simulink model "Duke_Simulink_13a"  (R2013a)
settings: Solver=FixedStepDiscrete  StartTime=0  StopTime=tempoSimulacao  FixedStep=1  RelTol=1e-3
values from neighbouring files (symbols this model uses):
  Ajustes_Inicial = dadosNumeroConstantes(linha)    [read_parametros_v2.m]
  aliquotaIR = dadosNumeroConstantes(linha)    [read_parametros_v2.m]
  CaixaInicial = dadosNumeroConstantes(linha)    [read_parametros_v2.m]
  Capital_Social_Inicial = CapitalSocial(1,2:end)    [Duke_main_v2.m]
  CFURH = dadosNumeroConstantes(linha)*TAR    [read_parametros_v2.m]
  contribuicaoCCEE = dadosNumeroConstantes(linha)    [read_parametros_v2.m]
  deducaoP_D = dadosNumeroConstantes(linha)    [read_parametros_v2.m]
  den_Ajustes = [1 zeros(1,PeriodoDepreciacao_Ajustes)]    [gera_Input_modelo.m]
  den_CustoAnual = [1 zeros(1,PeriodoCustoAnual-1)]    [gera_Input_modelo.m]
  den_CustoSemestral = [1 zeros(1,PeriodoCustoSemestral-1)]    [gera_Input_modelo.m]
  den_PPE_Edificacoes = [1 zeros(1,PPE_Periodo_Edificacoes)]    [gera_Input_modelo.m]
  den_PPE_Maquinas = [1 zeros(1,PPE_Periodo_Maquinas)]    [gera_Input_modelo.m]
  den_PPE_Moveis = [1 zeros(1,PPE_Periodo_Moveis)]    [gera_Input_modelo.m]
  den_PPE_Reservatorio = [1 zeros(1,PPE_Periodo_Reservatorio)]    [gera_Input_modelo.m]
  den_PPE_Veiculos = [1 zeros(1,PPE_Periodo_Veiculos)]    [gera_Input_modelo.m]
  DividaInicial = MtM_Total_Dividas(1,2:end)    [Duke_main_v2.m]
  Dividendos_A_Pagar_Inicial = dadosNumeroConstantes(linha)    [read_parametros_v2.m]
  garantiaFisica = dadosNumeroConstantes(linha)    [read_parametros_v2.m]
  IC_DividendosAPagarInicial = [repmat(vetor_DividendosAPagarInicial(1),numRealidades,1); zeros(realidadesPorSimulacao-numRealidades,1)]    [gera_Input_modelo.m]
  inicializa_JSCP = zeros(realidadesPorSimulacao,mes_JSCP)    [Duke_main_v2.m]
  IR_diferido_acumulado_inicial = dadosNumeroConstantes(linha)    [read_parametros_v2.m]
  JSCP_A_Pagar_Inicial = dadosNumeroConstantes(linha)    [read_parametros_v2.m]
  JSCP_ParcialPeriodo = dadosNumeroConstantes(linha)    [read_parametros_v2.m]
  JSCP_RetidoInicial = 0    [Duke_main_v2.m]
  Limite_Reserva_Lucros = dadosNumeroConstantes(linha)    [read_parametros_v2.m]
  Limite_Reserva_Lucros_Capital = dadosNumeroConstantes(linha)    [read_parametros_v2.m]
  LucroParcialPeriodo = dadosNumeroConstantes(linha)    [read_parametros_v2.m]
  LucroRetidoInicial = dadosNumeroConstantes(linha)    [read_parametros_v2.m]
  mes_DataInicial = month(DataInicial)    [Duke_main_v2.m]
  mes_JSCP = dadosNumeroConstantes(linha)    [read_parametros_v2.m]
  num_Ajustes = [0 ones(1,PeriodoDepreciacao_Ajustes)]*(1/PeriodoDepreciacao_Ajustes)    [gera_Input_modelo.m]
  num_CustoAnual = ones(1,PeriodoCustoAnual)*(1/PeriodoCustoAnual)    [gera_Input_modelo.m]
  num_CustoSemestral = ones(1,PeriodoCustoSemestral)*(1/PeriodoCustoSemestral)    [gera_Input_modelo.m]
  num_PPE_Edificacoes = [0 ones(1,PPE_Periodo_Edificacoes)]*(1/PPE_Periodo_Edificacoes)    [gera_Input_modelo.m]
  num_PPE_Maquinas = [0 ones(1,PPE_Periodo_Maquinas)]*(1/PPE_Periodo_Maquinas)    [gera_Input_modelo.m]
  num_PPE_Moveis = [0 ones(1,PPE_Periodo_Moveis)]*(1/PPE_Periodo_Moveis)    [gera_Input_modelo.m]
  num_PPE_Reservatorio = [0 ones(1,PPE_Periodo_Reservatorio)]*(1/PPE_Periodo_Reservatorio)    [gera_Input_modelo.m]
  num_PPE_Veiculos = [0 ones(1,PPE_Periodo_Veiculos)]*(1/PPE_Periodo_Veiculos)    [gera_Input_modelo.m]
  Outros_Passivos = dadosNumeroConstantes(linha)    [read_parametros_v2.m]
  periodoDividendos = dadosNumeroConstantes(linha)    [read_parametros_v2.m]
  periodoDividendos_delay = periodoDividendos    [Duke_main_v2.m]
  PeriodoIR_diferido = 12    [Duke_main_v2.m]
  PeriodoJSCP = 12    [Duke_main_v2.m]
  PIS_COFINS_Cumulativo = PIS + COFINS    [read_parametros_v2.m]
  PPE_Inicial_Edificacoes = dadosNumeroConstantes(linha)    [read_parametros_v2.m]
  PPE_Inicial_Maquinas = dadosNumeroConstantes(linha)    [read_parametros_v2.m]
  PPE_Inicial_Moveis = dadosNumeroConstantes(linha)    [read_parametros_v2.m]
  PPE_Inicial_Reservatorio = dadosNumeroConstantes(linha)    [read_parametros_v2.m]
  PPE_Inicial_Terreno = dadosNumeroConstantes(linha)    [read_parametros_v2.m]
  PPE_Inicial_Veiculos = dadosNumeroConstantes(linha)    [read_parametros_v2.m]
  refInd = (1-TEIFref)*(1-TEIPref)    [read_parametros_v2.m]
  Reserva_Capital_Inicial = dadosNumeroConstantes(linha)    [read_parametros_v2.m]
  Reserva_Lucros_Inicial = dadosNumeroConstantes(linha)    [read_parametros_v2.m]
  Taxa_Anual_Reserva = dadosNumeroConstantes(linha)    [read_parametros_v2.m]
  Taxa_diferimento = dadosNumeroConstantes(linha)    [read_parametros_v2.m]
  taxaMinorityInterest = dadosNumeroConstantes(linha)    [read_parametros_v2.m]
  TEIFa = dadosNumeroConstantes(linha)    [read_parametros_v2.m]
  TEIP = dadosNumeroConstantes(linha)    [read_parametros_v2.m]
  tempoSimulacao = 180    [Duke_main_v2.m]
  TEO = dadosNumeroConstantes(linha)    [read_parametros_v2.m]
  vetor_DividendosAPagarInicial = [repmat(vetor_DividendosAPagarInicial,numRealidades,1); zeros(realidadesPorSimulacao-numRealidades,periodoDividendos)]    [gera_Input_modelo.m]
  vetor_JSCP_APagarInicial = [repmat(vetor_JSCP_APagarInicial,numRealidades,1); zeros(realidadesPorSimulacao-numRealidades,PeriodoJSCP)]    [gera_Input_modelo.m]
undefined symbols (not defined in the file or in its folder): aDeducaoICMS, DiaPgtDespesasAdm, DiscIntNeverNeededParam, dts, IC_JSCP_APagarInicial, juros_ContasAPagar, juros_ContasAReceber, Media_DeprPPE, mediaADeducaoICMS, mediaADeducaoPISCOFINS, mediaRuidoGeracao, mediaTEIFa, mediaTEIP, Parametros, Periodo_Mes, PPE_Inicial, r, ruidoGeracaoSeed, Seed_DeprPPE, seedADeducaoICMS, seedADeducaoPISCOFINS, TEIFaSeed, TEIPSeed, Var_DeprPPE, varianciaADeducaoICMS, varianciaADeducaoPISCOFINS, varianciaRuidoGeracao, varianciaTEIFa, varianciaTEIP
libraries: simulink x22, dspsrcs4 x12
(part 2 of 2)

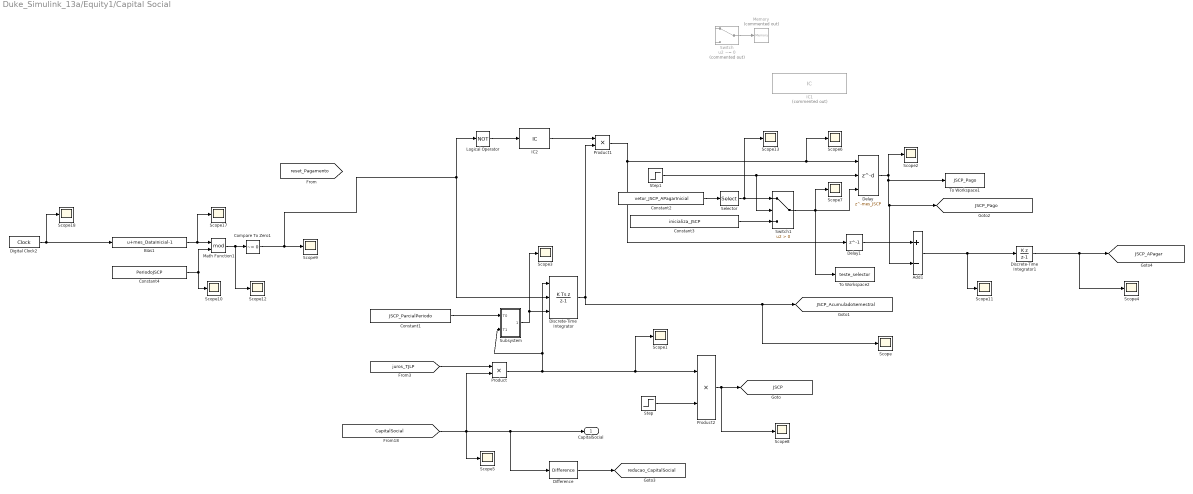
== system Duke_Simulink_13a/Equity1/Capital Social ==
  Add1 : Sum  Inputs=+-
  Bias1 : Bias  Bias=mes_DataInicial-1  SaturateOnIntegerOverflow=on
  Compare To Zero1 : simulink/Logic and Bit Operations/Compare To Zero  relop=~=  OutDataTypeStr=boolean
  Constant1 : Constant  Value=JSCP_ParcialPeriodo
  Constant2 : Constant  Value=vetor_JSCP_APagarInicial
  Constant3 : Constant  Value=inicializa_JSCP
  Constant4 : Constant  Value=PeriodoJSCP
  Delay : Delay  DelayLength=mes_JSCP  InitialConditionSource=Input port  InitialCondition=0  ExternalReset=Rising  InputProcessing=Inherited
      settings: InputPortMap=u0,r5,p4
  Delay1 : Delay  DelayLength=1
  Difference : simulink/Discrete/Difference  ICPrevInput=Capital_Social_Inicial  InputProcessing=Inherited  OutMin=[]  OutMax=[]  OutDataType=fixdt(1, 16)  OutScaling=2^-10  DoSatur=off
  Digital Clock2 : DigitalClock
  Discrete-Time Integrator : DiscreteIntegrator  IntegratorMethod=Integration: Backward Euler  ExternalReset=rising  InitialConditionSource=external  ICPrevOutput=DiscIntNeverNeededParam  ICPrevScaledInput=DiscIntNeverNeededParam
  Discrete-Time Integrator1 : DiscreteIntegrator  IntegratorMethod=Accumulation: Backward Euler  InitialCondition=JSCP_RetidoInicial  ICPrevOutput=DiscIntNeverNeededParam  ICPrevScaledInput=DiscIntNeverNeededParam
  IC1 : InitialCondition  Commented=on  Value=IC_JSCP_APagarInicial
  IC2 : InitialCondition  Value=false
  Logical Operator : Logic  Operator=NOT  AllPortsSameDT=off  OutDataTypeStr=boolean
  Math Function1 : Math  Operator=mod  SaturateOnIntegerOverflow=on
  Memory : Memory  Commented=on  X0=JSCP_A_Pagar_Inicial
  Product : Product
  Product1 : Product
  Product2 : Product  RndMeth=Zero
  Scope{,1..13,17..18} (16 alike) : Scope
      Scope settings: YMin=0  YMax=65000  SaveName=ScopeData20
      Scope1 settings: SaveName=ScopeData21
      Scope10 settings: SaveName=ScopeData160
      Scope11 settings: SaveName=ScopeData105
      Scope12 settings: SaveName=ScopeData161
      Scope13 settings: YMin=0  YMax=65000  SaveName=ScopeData162
      Scope17 settings: SaveName=ScopeData157
      Scope18 settings: SaveName=ScopeData158
      Scope2 settings: YMin=0  YMax=65000  SaveName=ScopeData37
      Scope3 settings: SaveName=ScopeData106
      Scope4 settings: SaveName=ScopeData108
      Scope5 settings: SaveName=ScopeData109
      Scope6 settings: YMin=0  YMax=65000  SaveName=ScopeData114
      Scope7 settings: YMin=0  YMax=65000  SaveName=ScopeData115
      Scope8 settings: YMin=0  YMax=65000  SaveName=ScopeData145
      Scope9 settings: SaveName=ScopeData159
  Selector : Selector  NumberOfDimensions=2  InputPortWidth=3  IndexOptions=Select all,Index vector (dialog)  Indices=[1 3],1:mes_JSCP  OutputSizes=1,1
  Step : Step  SampleTime=1
  Step1 : Step  SampleTime=1
  Subsystem : Subsystem
  Switch : Switch  Commented=on  Criteria=u2 ~= 0
  Switch1 : Switch  Criteria=u2 > Threshold
  To Workspace1 : ToWorkspace  VariableName=JSCP_Pago  SampleTime=-1  SaveFormat=Timeseries
  To Workspace2 : ToWorkspace  VariableName=teste_selector  SampleTime=-1
  CapitalSocial : Outport
  tag scope: JSCP=global, JSCP_APagar=global, JSCP_AcumuladoSemestral=global, JSCP_Pago=global, reducao_CapitalSocial=global
  wires:
  [CapitalSocial] -> Scope5/1, Product/2, Difference/1, CapitalSocial/1
  [juros_TJLP] -> Product/1
  Product/1 -> Subsystem/2(T1), Discrete-Time Integrator/1, Product2/1, Scope1/1
  Logical Operator/1 -> IC2/1
  Compare To Zero1/1 -> Discrete-Time Integrator/2, Logical Operator/1, Scope9/1
  Delay/1 -> Add1/2, [JSCP_Pago], To Workspace1/1, Scope2/1
  Step/1 -> Product2/2
  Product2/1 -> Scope8/1, [JSCP]
  Discrete-Time Integrator/1 -> Product1/2, [JSCP_AcumuladoSemestral], Scope/1
  Subsystem/1(Out1) -> Scope3/1, Discrete-Time Integrator/3
  Constant1/1 -> Subsystem/1(T0)
  IC2/1 -> Product1/1
  Product1/1 -> Delay1/1, Delay/1, Scope6/1
  Switch/1 -> Memory/1
  Discrete-Time Integrator1/1 -> Scope4/1, [JSCP_APagar]
  Difference/1 -> [reducao_CapitalSocial]
  Add1/1 -> Discrete-Time Integrator1/1, Scope11/1
  Delay1/1 -> Add1/1
  Digital Clock2/1 -> Scope18/1, Bias1/1
  Constant4/1 -> Scope10/1, Math Function1/2
  Math Function1/1 -> Scope12/1, Compare To Zero1/1
  Bias1/1 -> Scope17/1, Math Function1/1
  Switch1/1 -> To Workspace2/1, Delay/3, Scope7/1
  Constant2/1 -> Selector/1
  Step1/1 -> Delay/2, Switch1/2
  Selector/1 -> Scope13/1, Switch1/1
  Constant3/1 -> Switch1/3

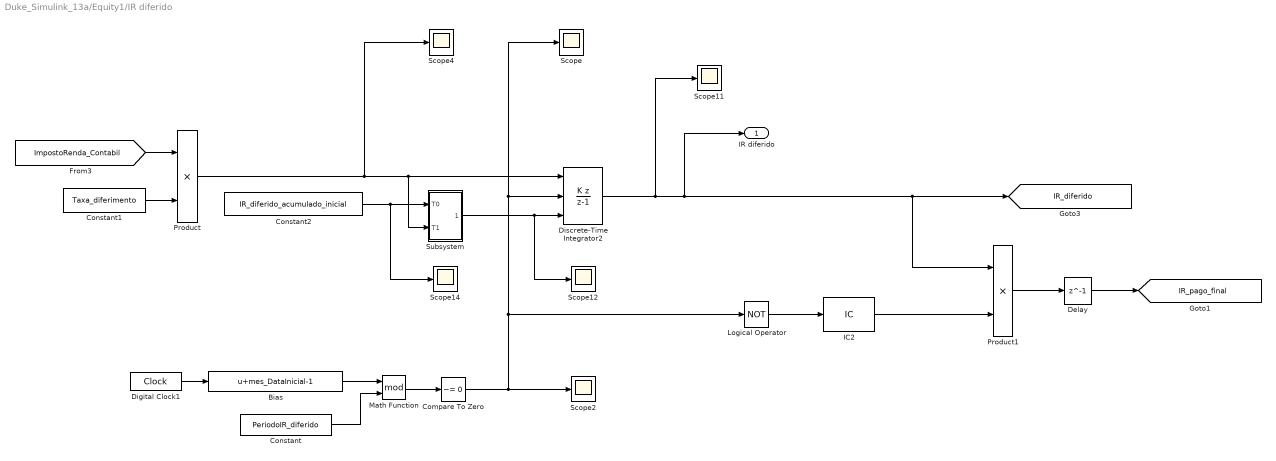
== system Duke_Simulink_13a/Equity1/IR diferido ==
  Bias : Bias  Bias=mes_DataInicial-1  SaturateOnIntegerOverflow=on
  Compare To Zero : simulink/Logic and Bit Operations/Compare To Zero  relop=~=  OutDataTypeStr=boolean
  Constant : Constant  Value=PeriodoIR_diferido
  Constant1 : Constant  Value=Taxa_diferimento
  Constant2 : Constant  Value=IR_diferido_acumulado_inicial
  Delay : Delay  DelayLength=1
  Digital Clock1 : DigitalClock
  Discrete-Time Integrator2 : DiscreteIntegrator  IntegratorMethod=Accumulation: Backward Euler  ExternalReset=rising  InitialConditionSource=external  ICPrevOutput=DiscIntNeverNeededParam  ICPrevScaledInput=DiscIntNeverNeededParam
  IC2 : InitialCondition  Value=false
  Logical Operator : Logic  Operator=NOT  AllPortsSameDT=off  OutDataTypeStr=boolean
  Math Function : Math  Operator=mod  SaturateOnIntegerOverflow=on
  Product : Product
  Product1 : Product
  Scope{,2,4,11,14} (5 alike) : Scope
      Scope settings: SaveName=ScopeData120
      Scope11 settings: SaveName=ScopeData104
      Scope14 settings: SaveName=ScopeData122
      Scope2 settings: SaveName=ScopeData124
      Scope4 settings: SaveName=ScopeData123
  "Scope12  " : Scope
      settings: SaveName=ScopeData121
  Subsystem : Subsystem
  IR diferido : Outport
  tag scope: IR_diferido=global, IR_pago_final=global
  wires:
  [ImpostoRenda_Contabil] -> Product/1
  Constant1/1 -> Product/2
  Discrete-Time Integrator2/1 -> Product1/1, [IR_diferido], IR diferido/1, Scope11/1
  Product/1 -> Scope4/1, Subsystem/2(T1), Discrete-Time Integrator2/1
  Constant2/1 -> Scope14/1, Subsystem/1(T0)
  Subsystem/1(Out1) -> "Scope12  "/1, Discrete-Time Integrator2/3
  Compare To Zero/1 -> Scope2/1, Logical Operator/1, Scope/1, Discrete-Time Integrator2/2
  Digital Clock1/1 -> Bias/1
  Constant/1 -> Math Function/2
  Math Function/1 -> Compare To Zero/1
  Bias/1 -> Math Function/1
  Logical Operator/1 -> IC2/1
  IC2/1 -> Product1/2
  Product1/1 -> Delay/1
  Delay/1 -> [IR_pago_final]

== system Duke_Simulink_13a/Equity1/Lucro Retido Total ==
  Add : Sum  Inputs=++++
  Scope{1..4,11} (5 alike) : Scope
      Scope1 settings: SaveName=ScopeData140
      Scope11 settings: SaveName=ScopeData104
      Scope2 settings: SaveName=ScopeData141
      Scope3 settings: SaveName=ScopeData142
      Scope4 settings: SaveName=ScopeData143
  Lucro Retido : Outport
  tag scope: Lucro_Retido_Total=global
  wires:
  [LucroAcumSemestral] -> Scope1/1, Add/1
  Add/1 -> Scope11/1, Lucro Retido/1, [Lucro_Retido_Total]
  [Lucro_Retido] -> Scope3/1, Add/3
  [JSCP_AcumuladoSemestral] -> Scope2/1, Add/2
  [JSCP_APagar] -> Scope4/1, Add/4

== system Duke_Simulink_13a/Equity1/Reserva ==
  Constant1 : Constant  Value=Taxa_Anual_Reserva
  Constant2 : Constant  Value=Reserva_Lucros_Inicial
  Constant3 : Constant  Value=Reserva_Capital_Inicial
  Difference : simulink/Discrete/Difference  ICPrevInput=Reserva_Lucros_Inicial  InputProcessing=Inherited  OutMin=[]  OutMax=[]  OutDataType=fixdt(1, 16)  OutScaling=2^-10  DoSatur=off
  Discrete-Time Integrator : DiscreteIntegrator  IntegratorMethod=Accumulation: Backward Euler  InitialConditionSource=external  ICPrevOutput=DiscIntNeverNeededParam  ICPrevScaledInput=DiscIntNeverNeededParam
  MinMax : MinMax  Inputs=2
  Product : Product
  Saturation : Saturate  UpperLimit=Limite_Reserva_Lucros*Capital_Social_Inicial  LowerLimit=0
  Saturation1 : Saturate  UpperLimit=Limite_Reserva_Lucros_Capital*Capital_Social_Inicial  LowerLimit=0
  Scope : Scope
      settings: SaveName=ScopeData85
  Sum : Sum
  Sum1 : Sum
  Sum2 : Sum  Inputs=-+
  Reserva Lucro e Capital : Outport
  tag scope: Reserva=global, Reserva_Lucros_fluxo=global
  wires:
  [Lucro_Liquido] -> Product/1
  Constant1/1 -> Product/2
  Constant2/1 -> Discrete-Time Integrator/2
  Discrete-Time Integrator/1 -> Sum/1, Saturation/1
  Product/1 -> Discrete-Time Integrator/1
  Difference/1 -> Scope/1, [Reserva_Lucros_fluxo]
  Sum/1 -> Saturation1/1
  Constant3/1 -> Sum2/1, Sum1/2, Sum/2
  Saturation1/1 -> MinMax/2
  Saturation/1 -> Sum1/1
  Sum1/1 -> MinMax/1
  MinMax/1 -> [Reserva], Reserva Lucro e Capital/1, Sum2/2
  Sum2/1 -> Difference/1

== system Duke_Simulink_13a/Equity1/Total Shareholder's Equity ==
  in : Inport
  out : Outport
  tag scope: TotalShareholdersEquity=global
  wires:
  in/1 -> [TotalShareholdersEquity], out/1

== system Duke_Simulink_13a/Income Statement/Acumulador8 ==
  In1 : Inport
  Discrete-Time Integrator1 : DiscreteIntegrator  IntegratorMethod=Accumulation: Backward Euler  InitialConditionSource=external  ICPrevOutput=DiscIntNeverNeededParam  ICPrevScaledInput=DiscIntNeverNeededParam
  Discrete-Time Integrator2 : DiscreteIntegrator  IntegratorMethod=Accumulation: Backward Euler  ICPrevOutput=DiscIntNeverNeededParam  ICPrevScaledInput=DiscIntNeverNeededParam
  Out1 : Outport
  wires:
  In1/1 -> Discrete-Time Integrator2/1
  Discrete-Time Integrator2/1 -> Out1/1

== system Duke_Simulink_13a/Income Statement/Amostrador6 ==
  In1 : Inport
  Gain1 : Gain  SampleTime=dts
  Out1 : Outport
  wires:
  In1/1 -> Gain1/1
  Gain1/1 -> Out1/1

== system Duke_Simulink_13a/Income Statement/Deduções Operacionais ==
  Add : Sum  Commented=on
  Add1 : Sum
  Add2 : Sum
  From Workspace1 : FromWorkspace  Commented=on  VariableName=PIS_COFINS_ICMS_Contratos_Total  SampleTime=1  Interpolate=off  OutputAfterFinalValue=Setting to zero
  ICMS : RandomNumber  Commented=on  Mean=mediaADeducaoICMS  Variance=varianciaADeducaoICMS  Seed=seedADeducaoICMS  SampleTime=1
  "ICMS " : Constant  Commented=on  Value=aDeducaoICMS
  PIS/COFINS : RandomNumber  Commented=on  Mean=mediaADeducaoPISCOFINS  Variance=varianciaADeducaoPISCOFINS  Seed=seedADeducaoPISCOFINS  SampleTime=1
  "PIS/COFINS " : Constant  Value=PIS_COFINS_Cumulativo
  Product1 : Product
  Scope1 : Scope
      settings: SaveName=ScopeData26
  Scope2 : Scope
      settings: SaveName=ScopeData33
  Scope6 : Scope
      settings: SaveName=ScopeData17
  deducoes : Outport
  wires:
  PIS/COFINS/1 -> Add/1
  ICMS/1 -> Add/2
  Add/1 -> ?
  [vendaSpot] -> Add2/1
  [vendaMRE_externo] -> Add2/2
  Add2/1 -> Product1/1
  "PIS/COFINS "/1 -> Product1/2, Scope6/1
  Add1/1 -> deducoes/1
  [PIS_COFINS_ICMS_Contratos_Total] -> Scope2/1, Add1/1
  Product1/1 -> Scope1/1, Add1/2

== system Duke_Simulink_13a/Income Statement/Depreciacao ==
  Depreciação : Outport
  wires:
  [Depreciacao] -> Depreciação/1

== system Duke_Simulink_13a/Income Statement/Despesas (Vendas, Gerais, Administrativas) ==
  Product1 : Product
  Product3 : Product
  Scope{1..4,6..8} (7 alike) : Scope
      Scope1 settings: SaveName=ScopeData70
      Scope2 settings: SaveName=ScopeData75
      Scope3 settings: SaveName=ScopeData76
      Scope4 settings: SaveName=ScopeData86
      Scope6 settings: SaveName=ScopeData91
      Scope7 settings: SaveName=ScopeData41
      Scope8 settings: SaveName=ScopeData42
  Total1 : Sum  Inputs=+|+
  Total2 : Sum  Inputs=+|+|+|+|+|+
  Total3 : Sum  Inputs=+|+
  Despesas : Outport
  wires:
  Total2/1 -> Despesas/1
  [compraMRE_externo] -> Scope8/1, Total2/4
  [compraSpot] -> Total2/3, Scope7/1
  [modeloIGPM] -> Scope4/1, Product1/2
  Total3/1 -> Scope3/1, Product1/1
  Product1/1 -> Total2/6
  Total1/1 -> Product3/1
  Product3/1 -> Scope6/1, Total2/5
  [curvaReajuste] -> Product3/2
  [AeG_labor] -> Total1/1
  [OeM_labor] -> Total1/2
  [AeG_expenses] -> Total3/1
  [OeM_expenses] -> Total3/2
  [regulatoryFees] -> Scope1/1, Total2/1
  [propertyAndOtherTaxes] -> Scope2/1, Total2/2

== system Duke_Simulink_13a/Income Statement/Despesas Financeiras ==
  note: Verificar se no mes que paga, o nonCash é oq incidiu naquele mes
  Distribuição CustoAnual1 : Subsystem
  Distribuição CustoSemestral : Subsystem
  Scope1 : Scope
      settings: SaveName=ScopeData173
  Scope11 : Scope
      settings: SaveName=ScopeData110
  Total4 : Sum  Inputs=---------
  Despesas Financeiras : Outport
  wires:
  [PnLPassivosLongoPrazoNonCash] -> Scope11/1, Total4/1
  Total4/1 -> Despesas Financeiras/1
  [Premio_PrePagamento] -> Scope1/1, Total4/3
  [otherInterestExpenses] -> Total4/2
  [Premio_ReducaoCapital_distribuido] -> Total4/4
  [CustoEmissao_distribuido] -> Total4/5
  [CustoCETIP] -> Total4/6
  [CustoMensal] -> Total4/7
  Distribuição CustoSemestral/1(CustoSemestral_Distribuido) -> Total4/8
  Distribuição CustoAnual1/1(CustoAnual_Distribuido) -> Total4/9

== system Duke_Simulink_13a/Income Statement/Earnings Before Financial Revenues // Expenses, Depreciation and Amortization ("EBITDA") (Lucro Operacional) ==
  in : Inport
  out : Outport
  wires:
  in/1 -> out/1

== system Duke_Simulink_13a/Income Statement/Earnings Before Financial Revenues and Expenses ("EBIT") ==
  in : Inport
  out : Outport
  wires:
  in/1 -> out/1

== system Duke_Simulink_13a/Income Statement/Imposto de Renda ==
  In1 : Inport
  Gain : Gain  Gain=aliquotaIR
  Saturation : Saturate  UpperLimit=Inf  LowerLimit=0
  Total5 : Sum  Inputs=+|+
  out : Outport
  wires:
  In1/1 -> Saturation/1
  Gain/1 -> Total5/1
  Saturation/1 -> Gain/1
  Total5/1 -> out/1
  [deferredIncomeTaxes] -> Total5/2

== system Duke_Simulink_13a/Income Statement/Lucro Liquido  ==
  in : Inport
  Add : Sum  Inputs=+-
  Constant : Constant  Value=taxaMinorityInterest
  Product : Product
  out : Outport
  tag scope: minorityInterest=global
  wires:
  Add/1 -> out/1
  in/1 -> Product/1, Add/1
  Constant/1 -> Product/2
  Product/1 -> Add/2, [minorityInterest]

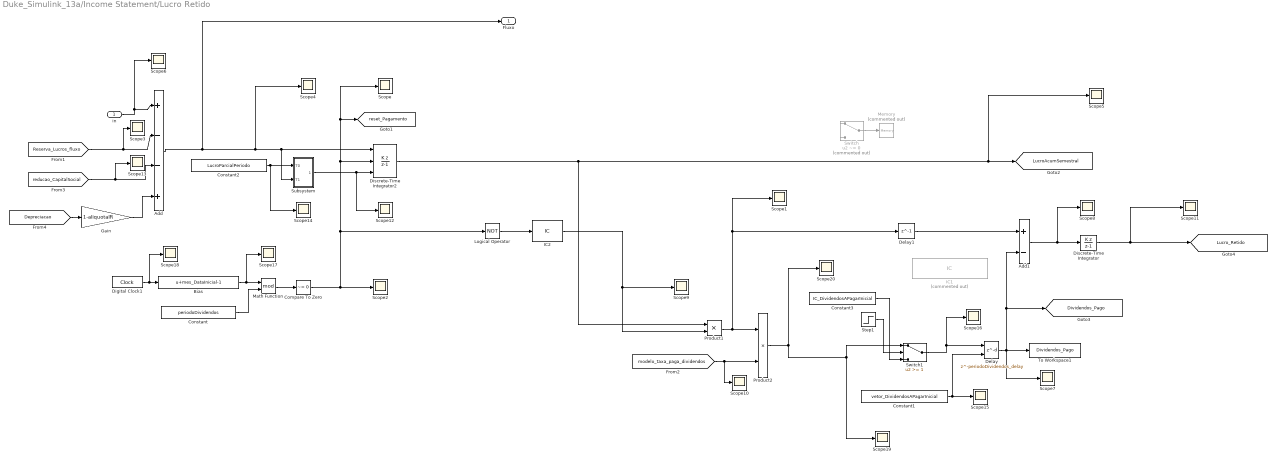
== system Duke_Simulink_13a/Income Statement/Lucro Retido ==
  in : Inport
  Add : Sum  Inputs=+--+
  Add1 : Sum  Inputs=+-
  Bias : Bias  Bias=mes_DataInicial-1  SaturateOnIntegerOverflow=on
  Compare To Zero : simulink/Logic and Bit Operations/Compare To Zero  relop=~=  OutDataTypeStr=boolean
  Constant : Constant  Value=periodoDividendos
  Constant1 : Constant  Value=vetor_DividendosAPagarInicial  OutDataTypeStr=double
  Constant2 : Constant  Value=LucroParcialPeriodo
  Constant3 : Constant  Value=IC_DividendosAPagarInicial
  Delay : Delay  DelayLength=periodoDividendos_delay  InitialConditionSource=Input port  InitialCondition=0  InputProcessing=Inherited
      settings: InputPortMap=u0,p4
  Delay1 : Delay  DelayLength=1
  Digital Clock1 : DigitalClock
  Discrete-Time Integrator : DiscreteIntegrator  IntegratorMethod=Accumulation: Backward Euler  InitialCondition=LucroRetidoInicial  ICPrevOutput=DiscIntNeverNeededParam  ICPrevScaledInput=DiscIntNeverNeededParam
  Discrete-Time Integrator2 : DiscreteIntegrator  IntegratorMethod=Accumulation: Backward Euler  ExternalReset=rising  InitialConditionSource=external  ICPrevOutput=DiscIntNeverNeededParam  ICPrevScaledInput=DiscIntNeverNeededParam
  Gain : Gain  Gain=1-aliquotaIR
  IC1 : InitialCondition  Commented=on  Value=IC_DividendosAPagarInicial
  IC2 : InitialCondition  Value=false
  Logical Operator : Logic  Operator=NOT  AllPortsSameDT=off  OutDataTypeStr=boolean
  Math Function : Math  Operator=mod  SaturateOnIntegerOverflow=on
  Memory : Memory  Commented=on  X0=Dividendos_A_Pagar_Inicial
  Product1 : Product
  Product2 : Product  RndMeth=Zero
  Scope{,1..20} (21 alike) : Scope
      Scope settings: SaveName=ScopeData22
      Scope1 settings: YMin=0  YMax=65000  SaveName=ScopeData18
      Scope10 settings: YMin=0  YMax=65000  SaveName=ScopeData102
      Scope11 settings: SaveName=ScopeData103
      Scope12 settings: SaveName=ScopeData107
      Scope13 settings: SaveName=ScopeData112
      Scope14 settings: SaveName=ScopeData113
      Scope15 settings: YMin=0  YMax=65000  SaveName=ScopeData116
      Scope16 settings: YMin=0  YMax=65000  SaveName=ScopeData117
      Scope17 settings: SaveName=ScopeData155
      Scope18 settings: SaveName=ScopeData156
      Scope19 settings: YMin=0  YMax=65000  SaveName=ScopeData165
      Scope2 settings: SaveName=ScopeData38
      Scope20 settings: YMin=0  YMax=65000  SaveName=ScopeData166
      Scope3 settings: SaveName=ScopeData44
      Scope4 settings: SaveName=ScopeData35
      Scope5 settings: SaveName=ScopeData39
      Scope6 settings: SaveName=ScopeData45
      Scope7 settings: TimeRange=600  YMin=0  YMax=1400000000  SaveName=ScopeData99
      Scope8 settings: YMin=0  YMax=65000  SaveName=ScopeData100
      Scope9 settings: YMin=0  YMax=65000  SaveName=ScopeData101
  Step1 : Step  SampleTime=1
  Subsystem : Subsystem
  Switch : Switch  Commented=on  Criteria=u2 ~= 0
  Switch1 : Switch  Threshold=1  OutDataTypeStr=double
  To Workspace1 : ToWorkspace  VariableName=Dividendos_Pago  SampleTime=-1  SaveFormat=Timeseries
  Fluxo : Outport
  tag scope: Dividendos_Pago=global, LucroAcumSemestral=global, Lucro_Retido=global, reset_Pagamento=global
  wires:
  in/1 -> Scope6/1, Add/1
  [Reserva_Lucros_fluxo] -> Scope3/1, Add/2
  Compare To Zero/1 -> Scope/1, [reset_Pagamento], Discrete-Time Integrator2/2, Logical Operator/1, Scope2/1
  Digital Clock1/1 -> Scope18/1, Bias/1
  Constant/1 -> Math Function/2
  Math Function/1 -> Compare To Zero/1
  Product1/1 -> Product2/1, Delay1/1, Scope1/1
  Logical Operator/1 -> IC2/1
  Add/1 -> Scope4/1, Subsystem/2(T1), Discrete-Time Integrator2/1, Fluxo/1
  [modelo_taxa_paga_dividendos] -> Scope10/1, Product2/2
  Bias/1 -> Scope17/1, Math Function/1
  Delay/1 -> Add1/2, [Dividendos_Pago], To Workspace1/1, Scope7/1
  Discrete-Time Integrator2/1 -> Scope5/1, [LucroAcumSemestral], Product1/1
  Constant2/1 -> Scope14/1, Subsystem/1(T0)
  Switch/1 -> Memory/1
  Constant1/1 -> Delay/2, Scope15/1
  Switch1/1 -> Scope16/1, Delay/1
  IC2/1 -> Scope9/1, Product1/2
  Subsystem/1(Out1) -> Scope12/1, Discrete-Time Integrator2/3
  Discrete-Time Integrator/1 -> Scope11/1, [Lucro_Retido]
  [reducao_CapitalSocial] -> Add/3, Scope13/1
  Step1/1 -> Switch1/2
  Constant3/1 -> Switch1/3
  [Depreciacao] -> Gain/1
  Add1/1 -> Scope8/1, Discrete-Time Integrator/1
  Delay1/1 -> Add1/1
  Product2/1 -> Scope19/1, Switch1/1, Scope20/1
  Gain/1 -> Add/4

== system Duke_Simulink_13a/Income Statement/Lucro Tributavel (EBT) - JSCP ==
  in : Inport
  Add : Sum  Inputs=+-  SampleTime=1
  Scope1 : Scope
      settings: SaveName=ScopeData154
  Scope3 : Scope
      settings: SaveName=ScopeData30
  out : Outport
  wires:
  Add/1 -> Scope1/1, out/1
  in/1 -> Add/1
  [JSCP] -> Scope3/1, Add/2

== system Duke_Simulink_13a/Income Statement/Outras receitas ==
  Total4 : Sum  Inputs=+|+
  Outras receitas : Outport
  wires:
  [operatingIncome] -> Total4/1
  [otherIncome] -> Total4/2
  Total4/1 -> Outras receitas/1

== system Duke_Simulink_13a/Income Statement/Receita Líquida ==
  in : Inport
  P_D : Constant  Value=deducaoP_D
  Product : Product
  Subtract : Sum  Inputs=+-
  out : Outport
  wires:
  in/1 -> Product/1, Subtract/1
  P_D/1 -> Product/2
  Product/1 -> Subtract/2
  Subtract/1 -> out/1

== system Duke_Simulink_13a/Income Statement/Receita Operacional ==
  From1 : From  Commented=on  GotoTag=Contratos_Leiloes
  From5 : From  Commented=on  GotoTag=Outros_ReceitaBruta
  Scope : Scope
      settings: SaveName=ScopeData90
  Scope1 : Scope
      settings: SaveName=ScopeData111
  Total2 : Sum  Inputs=+++
  receitaOperacional : Outport
  wires:
  Total2/1 -> receitaOperacional/1
  [contratosVenda] -> Scope/1, Total2/1
  [vendaSpot] -> Scope1/1, Total2/2
  [vendaMRE_externo] -> Total2/3

== system Duke_Simulink_13a/Income Statement/Receitas financeiras ==
  Receitas financeiras : Outport
  wires:
  [PnLCashCashEquivs] -> Receitas financeiras/1

== system Duke_Simulink_13a/Operacional/Contratos ==
  From Workspace : FromWorkspace  Commented=on  VariableName=energiaContratada_Total  SampleTime=1  Interpolate=off  OutputAfterFinalValue=Setting to zero
  From Workspace1 : FromWorkspace  Commented=on  VariableName=receitaContratada_Total  SampleTime=1  Interpolate=off  OutputAfterFinalValue=Setting to zero
  From Workspace2 : FromWorkspace  Commented=on  VariableName=vetor_horasMes  SampleTime=0
  Product : Product
  Scope1 : Scope
      settings: SaveName=ScopeData88
  Scope2 : Scope
      settings: SaveName=ScopeData87
  Energia Contratada : Outport
  Valor Contratado : Outport  Port=2
  wires:
  [receitaContratada_Total] -> Scope1/1, Valor Contratado/1
  [energiaContratada_Total] -> Product/1, Scope2/1
  [vetor_horasMes] -> Product/2
  Product/1 -> Energia Contratada/1

== system Duke_Simulink_13a/Operacional/Energia Alocada ==
  Constant : Constant  Commented=on  Value=TEIFa
  Constant1 : Constant  Commented=on  Value=TEIP
  FID : Subsystem  Commented=on
  From Workspace : FromWorkspace  Commented=on  VariableName=vetor_horasMes  SampleTime=0
  GSF : FromWorkspace  Commented=on  VariableName=modeloGSF  SampleTime=1  Interpolate=off  OutputAfterFinalValue=Setting to zero
  Garantia Física Sazonalizada : FromWorkspace  Commented=on  VariableName=modeloSazonalizacaoGF  SampleTime=1  Interpolate=off  OutputAfterFinalValue=Setting to zero
  Parada Forçada : RandomNumber  Commented=on  Mean=mediaTEIFa  Variance=varianciaTEIFa  Seed=TEIFaSeed  SampleTime=1
  Parada Programada : RandomNumber  Commented=on  Mean=mediaTEIP  Variance=varianciaTEIP  Seed=TEIPSeed  SampleTime=1
  Product : Product
  Product2 : Product  RndMeth=Zero
  Scope1 : Scope
  Scope3 : Scope
      settings: SaveName=ScopeData3
  To Workspace1 : ToWorkspace  Commented=on  VariableName=FID  SampleTime=1  SaveFormat=Timeseries
  Energia Alocada : Outport
  wires:
  Product2/1 -> Energia Alocada/1  "em MWh"
  FID/1(FID) -> To Workspace1/1
  Constant1/1 -> FID/2(TEIP)
  Constant/1 -> FID/1(TEIFa)
  [GF_sazonalizada] -> Product/1, Scope3/1
  [modeloGSF] -> Product2/1, Scope1/1
  [vetor_horasMes] -> Product/2
  Product/1 -> Product2/2

== system Duke_Simulink_13a/Operacional/Geração ==
  note: em R$/MWh
  Energia Alocada : Inport
  Add1 : Sum  Inputs=-+
  Add2 : Sum  Inputs=+-
  CCEE : Constant  Value=contribuicaoCCEE
  Energia gerada : RandomNumber  Commented=on  Mean=mediaRuidoGeracao  Variance=varianciaRuidoGeracao  Seed=ruidoGeracaoSeed  SampleTime=1
  From Workspace : FromWorkspace  Commented=on  VariableName=vetor_horasMes  SampleTime=0
  GF : Constant  Value=garantiaFisica
  Gain : Gain  Commented=on  Gain=0.001
  Gain1 : Gain  Gain=CFURH
  Product : Product
  Product1 : Product  RndMeth=Zero
  Product4 : Product  RndMeth=Zero
  Step : Step  SampleTime=1
  TEO : Constant  Value=TEO
  scope{,1..3} (4 alike) : Scope
      scope settings: SaveName=ScopeData92
      scope1 settings: SaveName=ScopeData93
      scope2 settings: SaveName=ScopeData94
      scope3 settings: SaveName=ScopeData95
  Valor MRE : Outport
  tag scope: royaltiesAgua=global
  wires:
  Energia Alocada/1 -> scope3/1, Add1/1  "em MWh"
  Add1/1 -> scope1/1, Product4/1  "em MWh"
  Product4/1 -> scope2/1, Valor MRE/1  "em R$"
  Gain1/1 -> [royaltiesAgua]  "em R$"
  TEO/1 -> Add2/1
  CCEE/1 -> Add2/2
  Add2/1 -> Product4/2  "em R$/MWh"
  Product1/1 -> scope/1, Add1/2, Gain1/1
  Step/1 -> Product1/2
  [vetor_horasMes] -> Product/2
  Product/1 -> Product1/1  "em MWh"
  GF/1 -> Product/1

== system Duke_Simulink_13a/Operacional/PLD ==
  From Workspace1 : FromWorkspace  Commented=on  VariableName=modeloPLD  SampleTime=1  Interpolate=off  OutputAfterFinalValue=Setting to zero
  Scope2 : Scope
      settings: SaveName=ScopeData2
  PLD : Outport
  wires:
  [modeloPLD] -> Scope2/1, PLD/1

== system Duke_Simulink_13a/Passivos1/Contas a Pagar ==
  Constant1 : Constant  Commented=on  Value=juros_ContasAPagar
  Modified Difference1 : Subsystem
  Product : Product
  Total5 : Sum  Inputs=+++++
  MtM1 : Outport
  tag scope: MtMContasPagar=global, PnLContasPagar=global, deltaMtMContasPagar=global
  wires:
  Product/1 -> [PnLContasPagar]
  Modified Difference1/1(Delta) -> [deltaMtMContasPagar]
  Total5/1 -> Product/1, [MtMContasPagar], Modified Difference1/1(In1), MtM1/1
  ? -> Product/2

== system Duke_Simulink_13a/Passivos1/Outros Passivos ==
  Constant : Constant  Commented=on  Value=Parametros.juros.PassivosNaoCirculantes
  Constant1 : Constant  Value=Outros_Passivos
  Modified Difference : Subsystem
  Product : Product
  MtM : Outport
  tag scope: MtMOutrosPassivos=global, PnLOutrosPassivosCash=global, PnLOutrosPassivosNonCash=global, deltaMtMOutrosPassivos=global
  wires:
  Constant1/1 -> Product/1, Modified Difference/1(In1), [MtMOutrosPassivos], MtM/1
  Modified Difference/1(Delta) -> [deltaMtMOutrosPassivos]
  Product/1 -> ?
  ? -> Product/2

== system Duke_Simulink_13a/Passivos1/Passivos de Curto Prazo ==
  note: Verificar em Lucro Retido
  Difference : simulink/Discrete/Difference  ICPrevInput=0.0  OutMin=[]  OutMax=[]  OutDataType=fixdt(1, 16)  OutScaling=2^-10  DoSatur=off
  Scope3 : Scope
      settings: SaveName=ScopeData98
  MtM : Outport
  tag scope: MtMPassivosCurtoPrazo=global, deltaMtMPassivosCurtoPrazo=global
  wires:
  [DebtPlug] -> [MtMPassivosCurtoPrazo], Difference/1, Scope3/1, MtM/1  "Passivo de Curto Prazo"
  Difference/1 -> [deltaMtMPassivosCurtoPrazo]

== system Duke_Simulink_13a/Passivos1/Passivos de Longo Prazo ==
  Difference : simulink/Discrete/Difference  ICPrevInput=DividaInicial  InputProcessing=Inherited  OutMin=[]  OutMax=[]  OutDataType=fixdt(1, 16)  OutScaling=2^-10  DoSatur=off
  Digital Clock : DigitalClock  Commented=on
  MtM de Todas Dividas : FromWorkspace  Commented=on  VariableName=MtM_Total_Dividas  SampleTime=1  Interpolate=off  OutputAfterFinalValue=Setting to zero
  Scope : Scope
      settings: SaveName=ScopeData25
  Scope3 : Scope
      settings: SaveName=ScopeData40
  Scope6 : Scope
      settings: SaveName=ScopeData43
  Sum5 : Sum
  MtM : Outport
  tag scope: MtMPassivosLongoPrazo=global, PnLPassivosLongoPrazo=global, PnLPassivosLongoPrazoCash=global, PnLPassivosLongoPrazoNonCash=global, deltaMtMPassivosLongoPrazo=global
  wires:
  Difference/1 -> Scope3/1, [deltaMtMPassivosLongoPrazo]
  [MtM_Total_Dividas] -> Difference/1, Scope/1, MtM/1, [MtMPassivosLongoPrazo]
  [PnLnonCash_Total_Dividas] -> [PnLPassivosLongoPrazoNonCash], Sum5/1
  [PnLCash_Total_Dividas] -> Sum5/2, [PnLPassivosLongoPrazoCash]
  Sum5/1 -> Scope6/1, [PnLPassivosLongoPrazo]

== system Duke_Simulink_13a/Passivos1/Total Passivos ==
  in : Inport
  out : Outport
  tag scope: TotalPassivos=global
  wires:
  in/1 -> [TotalPassivos], out/1

== system Duke_Simulink_13a/Passivos1/Total Passivos & Equity ==
  in : Inport
  out : Outport
  tag scope: TotalPassivosPlusEquity=global
  wires:
  in/1 -> out/1, [TotalPassivosPlusEquity]

== system Duke_Simulink_13a/Passivos1/Total Passivos de Curto Prazo ==
  in : Inport
  out : Outport
  tag scope: TotalPassivosCurtoPrazo=global
  wires:
  in/1 -> out/1, [TotalPassivosCurtoPrazo]

== system Duke_Simulink_13a/Ativos1/Contas a Receber (Recebíveis)/Amostrador1 ==
  In1 : Inport
  Constant : Constant
  Product : Product  SampleTime=1  RndMeth=Zero
  Out1 : Outport
  wires:
  Product/1 -> Out1/1
  In1/1 -> Product/1
  Constant/1 -> Product/2

== system Duke_Simulink_13a/Ativos1/Contas a Receber (Recebíveis)/Modified Difference ==
  In1 : Inport
  Difference : simulink/Discrete/Difference  ICPrevInput=0.0  OutMin=[]  OutMax=[]  OutDataType=fixdt(1, 16)  OutScaling=2^-10  DoSatur=off
  Discrete Impulse1 : dspsrcs4/Discrete  Impulse  Delay=0  SampleTime=1  FrameSample=1  dataType=double  isSigned=on  wordLen=16  udDataType=sfix(16)  fracBitsMode=Best precision  numFracBits=15  OutDataTypeStr=double  LastOutDataTypeStr=double
  Product3 : Product  RndMeth=Zero
  Total3 : Sum  Inputs=+-
  Delta : Outport
  wires:
  Total3/1 -> Delta/1
  In1/1 -> Product3/1, Difference/1
  Product3/1 -> Total3/2
  Discrete Impulse1/1 -> Product3/2
  Difference/1 -> Total3/1

== system Duke_Simulink_13a/Ativos1/Estoque/Amostrador1 ==
  In1 : Inport
  Gain1 : Gain  SampleTime=dts
  Out1 : Outport
  wires:
  Gain1/1 -> Out1/1
  In1/1 -> Gain1/1

== system Duke_Simulink_13a/Ativos1/Estoque/Modified Difference ==
  In1 : Inport
  Difference : simulink/Discrete/Difference  ICPrevInput=0.0  OutMin=[]  OutMax=[]  OutDataType=fixdt(1, 16)  OutScaling=2^-10  DoSatur=off
  Discrete Impulse1 : dspsrcs4/Discrete  Impulse  Delay=0  SampleTime=1  FrameSample=1  dataType=double  isSigned=on  wordLen=16  udDataType=sfix(16)  fracBitsMode=Best precision  numFracBits=15  OutDataTypeStr=double  LastOutDataTypeStr=double
  Product3 : Product  RndMeth=Zero
  Total3 : Sum  Inputs=+-
  Delta : Outport
  wires:
  Total3/1 -> Delta/1
  In1/1 -> Product3/1, Difference/1
  Product3/1 -> Total3/2
  Discrete Impulse1/1 -> Product3/2
  Difference/1 -> Total3/1

== system Duke_Simulink_13a/Ativos1/Financial Instruments (Hedging)/Modified Difference1 ==
  In1 : Inport
  Difference : simulink/Discrete/Difference  ICPrevInput=0.0  OutMin=[]  OutMax=[]  OutDataType=fixdt(1, 16)  OutScaling=2^-10  DoSatur=off
  Discrete Impulse1 : dspsrcs4/Discrete  Impulse  Delay=0  SampleTime=1  FrameSample=1  dataType=double  isSigned=on  wordLen=16  udDataType=sfix(16)  fracBitsMode=Best precision  numFracBits=15  OutDataTypeStr=double  LastOutDataTypeStr=double
  Product3 : Product  RndMeth=Zero
  Total3 : Sum  Inputs=+-
  Delta : Outport
  wires:
  In1/1 -> Product3/1, Difference/1
  Product3/1 -> Total3/2
  Discrete Impulse1/1 -> Product3/2
  Difference/1 -> Total3/1
  Total3/1 -> Delta/1

== system Duke_Simulink_13a/Ativos1/Net PP&E/Edificacoes ==
  Add1 : Sum
  Add2 : Sum
  Discrete Transfer Fcn : DiscreteTransferFcn  Numerator=num_PPE_Edificacoes  Denominator=den_PPE_Edificacoes  SampleTime=1
  Discrete Impulse : dspsrcs4/Discrete  Impulse  Delay=0  SampleTime=1  FrameSample=1  dataType=double  isSigned=on  wordLen=16  udDataType=sfix(16)  fracBitsMode=Best precision  numFracBits=15  OutDataTypeStr=double  LastOutDataTypeStr=double
  Discrete-Time Integrator6 : DiscreteIntegrator  IntegratorMethod=Accumulation: Backward Euler  InitialConditionSource=external  ICPrevOutput=DiscIntNeverNeededParam  ICPrevScaledInput=DiscIntNeverNeededParam
  Gain : Gain  Gain=-1
  Investimento Inicial19 : Constant  Value=PPE_Inicial_Edificacoes
  Product1 : Product
  Scope1 : Scope
      settings: SaveName=ScopeData67
  Depreciacao : Outport
  PPE : Outport  Port=2
  wires:
  Discrete Impulse/1 -> Product1/2
  Add1/1 -> Discrete Transfer Fcn/1
  Discrete Transfer Fcn/1 -> Gain/1, Depreciacao/1, Scope1/1
  Product1/1 -> Add1/1
  Investimento Inicial19/1 -> Discrete-Time Integrator6/2, Product1/1
  [PPE_Compras_Edificacoes] -> Add2/2, Add1/2
  Add2/1 -> Discrete-Time Integrator6/1
  Gain/1 -> Add2/1
  Discrete-Time Integrator6/1 -> PPE/1

== system Duke_Simulink_13a/Ativos1/Net PP&E/Maquinas ==
  Add1 : Sum
  Add2 : Sum
  Discrete Transfer Fcn : DiscreteTransferFcn  Numerator=num_PPE_Maquinas  Denominator=den_PPE_Maquinas  SampleTime=1
  Discrete Impulse : dspsrcs4/Discrete  Impulse  Delay=0  SampleTime=1  FrameSample=1  dataType=double  isSigned=on  wordLen=16  udDataType=sfix(16)  fracBitsMode=Best precision  numFracBits=15  OutDataTypeStr=double  LastOutDataTypeStr=double
  Discrete-Time Integrator6 : DiscreteIntegrator  IntegratorMethod=Accumulation: Backward Euler  InitialConditionSource=external  ICPrevOutput=DiscIntNeverNeededParam  ICPrevScaledInput=DiscIntNeverNeededParam
  Gain : Gain  Gain=-1
  Investimento Inicial19 : Constant  Value=PPE_Inicial_Maquinas
  Product1 : Product
  Scope1 : Scope
      settings: SaveName=ScopeData67
  Depreciacao : Outport
  PPE : Outport  Port=2
  wires:
  Discrete-Time Integrator6/1 -> PPE/1
  Gain/1 -> Add2/1
  Add2/1 -> Discrete-Time Integrator6/1
  [PPE_Compras_Maquinas] -> Add1/2, Add2/2
  Investimento Inicial19/1 -> Product1/1, Discrete-Time Integrator6/2
  Product1/1 -> Add1/1
  Discrete Transfer Fcn/1 -> Scope1/1, Depreciacao/1, Gain/1
  Add1/1 -> Discrete Transfer Fcn/1
  Discrete Impulse/1 -> Product1/2

== system Duke_Simulink_13a/Ativos1/Net PP&E/Moveis ==
  Add1 : Sum
  Add2 : Sum
  Discrete Transfer Fcn : DiscreteTransferFcn  Numerator=num_PPE_Moveis  Denominator=den_PPE_Moveis  SampleTime=1
  Discrete Impulse : dspsrcs4/Discrete  Impulse  Delay=0  SampleTime=1  FrameSample=1  dataType=double  isSigned=on  wordLen=16  udDataType=sfix(16)  fracBitsMode=Best precision  numFracBits=15  OutDataTypeStr=double  LastOutDataTypeStr=double
  Discrete-Time Integrator6 : DiscreteIntegrator  IntegratorMethod=Accumulation: Backward Euler  InitialConditionSource=external  ICPrevOutput=DiscIntNeverNeededParam  ICPrevScaledInput=DiscIntNeverNeededParam
  Gain : Gain  Gain=-1
  Investimento Inicial19 : Constant  Value=PPE_Inicial_Moveis
  Product1 : Product
  Scope1 : Scope
      settings: SaveName=ScopeData67
  Depreciacao : Outport
  PPE : Outport  Port=2
  wires:
  Discrete-Time Integrator6/1 -> PPE/1
  Gain/1 -> Add2/1
  Add2/1 -> Discrete-Time Integrator6/1
  [PPE_Compras_Moveis] -> Add1/2, Add2/2
  Investimento Inicial19/1 -> Product1/1, Discrete-Time Integrator6/2
  Product1/1 -> Add1/1
  Discrete Transfer Fcn/1 -> Scope1/1, Depreciacao/1, Gain/1
  Add1/1 -> Discrete Transfer Fcn/1
  Discrete Impulse/1 -> Product1/2

== system Duke_Simulink_13a/Ativos1/Net PP&E/Reservatorio ==
  Add1 : Sum
  Add2 : Sum
  Discrete Transfer Fcn : DiscreteTransferFcn  Numerator=num_PPE_Reservatorio  Denominator=den_PPE_Reservatorio  SampleTime=1
  Discrete Impulse : dspsrcs4/Discrete  Impulse  Delay=0  SampleTime=1  FrameSample=1  dataType=double  isSigned=on  wordLen=16  udDataType=sfix(16)  fracBitsMode=Best precision  numFracBits=15  OutDataTypeStr=double  LastOutDataTypeStr=double
  Discrete-Time Integrator6 : DiscreteIntegrator  IntegratorMethod=Accumulation: Backward Euler  InitialConditionSource=external  ICPrevOutput=DiscIntNeverNeededParam  ICPrevScaledInput=DiscIntNeverNeededParam
  Gain : Gain  Gain=-1
  Investimento Inicial19 : Constant  Value=PPE_Inicial_Reservatorio
  Product1 : Product
  Scope1 : Scope
      settings: SaveName=ScopeData67
  Depreciacao : Outport
  PPE : Outport  Port=2
  wires:
  Discrete-Time Integrator6/1 -> PPE/1
  Gain/1 -> Add2/1
  Add2/1 -> Discrete-Time Integrator6/1
  [PPE_Compras_Reservatorio] -> Add1/2, Add2/2
  Investimento Inicial19/1 -> Product1/1, Discrete-Time Integrator6/2
  Product1/1 -> Add1/1
  Discrete Transfer Fcn/1 -> Scope1/1, Depreciacao/1, Gain/1
  Add1/1 -> Discrete Transfer Fcn/1
  Discrete Impulse/1 -> Product1/2

== system Duke_Simulink_13a/Ativos1/Net PP&E/Terreno ==
  note: BLOCO ALTERADO
      | Terreno nao deprecia
  Add1 : Sum
  Add2 : Sum
  Discrete Transfer Fcn : DiscreteTransferFcn  Numerator=[0 ones(1,tempoSimulacao)]*0  Denominator=[1 zeros(1,tempoSimulacao)]  SampleTime=1
  Discrete Impulse : dspsrcs4/Discrete  Impulse  Delay=0  SampleTime=1  FrameSample=1  dataType=double  isSigned=on  wordLen=16  udDataType=sfix(16)  fracBitsMode=Best precision  numFracBits=15  OutDataTypeStr=double  LastOutDataTypeStr=double
  Discrete-Time Integrator6 : DiscreteIntegrator  IntegratorMethod=Accumulation: Backward Euler  InitialConditionSource=external  ICPrevOutput=DiscIntNeverNeededParam  ICPrevScaledInput=DiscIntNeverNeededParam
  Gain : Gain  Gain=-1
  Investimento Inicial1 : Constant  Value=PPE_Inicial_Terreno
  Product1 : Product
  Scope1 : Scope
      settings: SaveName=ScopeData67
  Depreciacao : Outport
  PPE : Outport  Port=2
  wires:
  Discrete Impulse/1 -> Product1/2
  Add1/1 -> Discrete Transfer Fcn/1
  Discrete Transfer Fcn/1 -> Gain/1, Depreciacao/1, Scope1/1
  Product1/1 -> Add1/1
  Investimento Inicial1/1 -> Discrete-Time Integrator6/2, Product1/1
  [PPE_Compras_Terreno] -> Add2/2, Add1/2
  Add2/1 -> Discrete-Time Integrator6/1
  Gain/1 -> Add2/1
  Discrete-Time Integrator6/1 -> PPE/1

== system Duke_Simulink_13a/Ativos1/Net PP&E/Veiculos ==
  Add1 : Sum
  Add2 : Sum
  Discrete Transfer Fcn : DiscreteTransferFcn  Numerator=num_PPE_Veiculos  Denominator=den_PPE_Veiculos  SampleTime=1
  Discrete Impulse : dspsrcs4/Discrete  Impulse  Delay=0  SampleTime=1  FrameSample=1  dataType=double  isSigned=on  wordLen=16  udDataType=sfix(16)  fracBitsMode=Best precision  numFracBits=15  OutDataTypeStr=double  LastOutDataTypeStr=double
  Discrete-Time Integrator6 : DiscreteIntegrator  IntegratorMethod=Accumulation: Backward Euler  InitialConditionSource=external  ICPrevOutput=DiscIntNeverNeededParam  ICPrevScaledInput=DiscIntNeverNeededParam
  Gain : Gain  Gain=-1
  Investimento Inicial19 : Constant  Value=PPE_Inicial_Veiculos
  Product1 : Product
  Scope1 : Scope
      settings: SaveName=ScopeData67
  Depreciacao : Outport
  PPE : Outport  Port=2
  wires:
  Discrete Impulse/1 -> Product1/2
  Add1/1 -> Discrete Transfer Fcn/1
  Discrete Transfer Fcn/1 -> Gain/1, Depreciacao/1, Scope1/1
  Product1/1 -> Add1/1
  Investimento Inicial19/1 -> Discrete-Time Integrator6/2, Product1/1
  [PPE_Compras_Veiculos] -> Add2/2, Add1/2
  Add2/1 -> Discrete-Time Integrator6/1
  Gain/1 -> Add2/1
  Discrete-Time Integrator6/1 -> PPE/1

== system Duke_Simulink_13a/Ativos1/Property, Plant & Equipment/Amostrador2 ==
  In1 : Inport
  Gain1 : Gain  SampleTime=dts
  Out1 : Outport
  wires:
  In1/1 -> Gain1/1
  Gain1/1 -> Out1/1

== system Duke_Simulink_13a/Equity1/Ajustes/Reservatorio ==
  Add1 : Sum
  Add2 : Sum
  Discrete Transfer Fcn : DiscreteTransferFcn  Numerator=num_Ajustes  Denominator=den_Ajustes  SampleTime=1
  Discrete Impulse : dspsrcs4/Discrete  Impulse  Delay=0  SampleTime=1  FrameSample=1  dataType=double  isSigned=on  wordLen=16  udDataType=sfix(16)  fracBitsMode=Best precision  numFracBits=15  OutDataTypeStr=double  LastOutDataTypeStr=double
  Discrete-Time Integrator6 : DiscreteIntegrator  IntegratorMethod=Accumulation: Backward Euler  InitialConditionSource=external  ICPrevOutput=DiscIntNeverNeededParam  ICPrevScaledInput=DiscIntNeverNeededParam
  Gain : Gain  Gain=-1
  Investimento Inicial19 : Constant  Value=Ajustes_Inicial
  Product1 : Product
  Scope1 : Scope
      settings: SaveName=ScopeData67
  Depreciacao : Outport
  PPE : Outport  Port=2
  wires:
  Discrete-Time Integrator6/1 -> PPE/1
  Gain/1 -> Add2/1
  Add2/1 -> Discrete-Time Integrator6/1
  [Ajustes_Adicionais] -> Add1/2, Add2/2
  Investimento Inicial19/1 -> Product1/1, Discrete-Time Integrator6/2
  Product1/1 -> Add1/1
  Discrete Transfer Fcn/1 -> Scope1/1, Depreciacao/1, Gain/1
  Add1/1 -> Discrete Transfer Fcn/1
  Discrete Impulse/1 -> Product1/2

== system Duke_Simulink_13a/Equity1/Capital Social/Subsystem ==
  T0 : Inport
  T1 : Inport  Port=2
  Product3 : Product  RndMeth=Zero
  Product4 : Product  RndMeth=Zero
  Step1 : Step  Before=1  After=0  SampleTime=1
  Step2 : Step  SampleTime=1
  Total5 : Sum  Inputs=+|+
  Out1 : Outport
  wires:
  T0/1 -> Product3/1
  Step1/1 -> Product3/2
  Total5/1 -> Out1/1
  Product3/1 -> Total5/1
  Product4/1 -> Total5/2
  Step2/1 -> Product4/2
  T1/1 -> Product4/1

== system Duke_Simulink_13a/Equity1/IR diferido/Subsystem ==
  T0 : Inport
  T1 : Inport  Port=2
  Product3 : Product  RndMeth=Zero
  Product4 : Product  RndMeth=Zero
  Step1 : Step  Before=1  After=0  SampleTime=1
  Step2 : Step  SampleTime=1
  Total5 : Sum  Inputs=+|+
  Out1 : Outport
  wires:
  T0/1 -> Product3/1
  Step1/1 -> Product3/2
  Total5/1 -> Out1/1
  Product3/1 -> Total5/1
  Product4/1 -> Total5/2
  Step2/1 -> Product4/2
  T1/1 -> Product4/1

== system Duke_Simulink_13a/Income Statement/Despesas Financeiras/Distribuição CustoAnual1 ==
  Discrete Transfer Fcn : DiscreteTransferFcn  Numerator=num_CustoAnual  Denominator=den_CustoAnual  SampleTime=1
  Scope1 : Scope
      settings: SaveName=ScopeData67
  Scope2 : Scope
      settings: TimeRange=180  YMin=0  YMax=400000  SaveName=ScopeData144
  CustoAnual_Distribuido : Outport
  wires:
  [CustoAnual] -> Discrete Transfer Fcn/1, Scope2/1
  Discrete Transfer Fcn/1 -> Scope1/1, CustoAnual_Distribuido/1

== system Duke_Simulink_13a/Income Statement/Despesas Financeiras/Distribuição CustoSemestral ==
  Discrete Transfer Fcn : DiscreteTransferFcn  Numerator=num_CustoSemestral  Denominator=den_CustoSemestral  SampleTime=1
  Scope1 : Scope
      settings: SaveName=ScopeData67
  Scope2 : Scope
      settings: TimeRange=180  YMin=0  YMax=400000  SaveName=ScopeData144
  CustoSemestral_Distribuido : Outport
  wires:
  Discrete Transfer Fcn/1 -> CustoSemestral_Distribuido/1, Scope1/1
  [CustoSemestral] -> Scope2/1, Discrete Transfer Fcn/1

== system Duke_Simulink_13a/Income Statement/Lucro Retido/Subsystem ==
  T0 : Inport
  T1 : Inport  Port=2
  Product3 : Product  RndMeth=Zero
  Product4 : Product  RndMeth=Zero
  Step1 : Step  Before=1  After=0  SampleTime=1
  Step2 : Step  SampleTime=1
  Total5 : Sum  Inputs=+|+
  Out1 : Outport
  wires:
  T0/1 -> Product3/1
  Step1/1 -> Product3/2
  Total5/1 -> Out1/1
  Product3/1 -> Total5/1
  Product4/1 -> Total5/2
  Step2/1 -> Product4/2
  T1/1 -> Product4/1

== system Duke_Simulink_13a/Operacional/Energia Alocada/FID ==
  TEIFa : Inport
  TEIP : Inport  Port=2
  Add : Sum  Inputs=+-
  Add1 : Sum  Inputs=+-
  Constant1 : Constant
  Constant2 : Constant
  Divide : Product  Inputs=*/
  Indisponibilidade de Referência : Constant  Value=refInd
  Product : Product  RndMeth=Zero
  Saturation : Saturate  UpperLimit=1  LowerLimit=0
  FID : Outport
  wires:
  TEIFa/1 -> Add/2
  Add/1 -> Product/1
  TEIP/1 -> Add1/2
  Constant2/1 -> Add1/1
  Divide/1 -> Saturation/1
  Product/1 -> Divide/1
  Add1/1 -> Product/2
  Indisponibilidade de Referência/1 -> Divide/2
  Constant1/1 -> Add/1
  Saturation/1 -> FID/1

== system Duke_Simulink_13a/Passivos1/Contas a Pagar/Modified Difference1 ==
  In1 : Inport
  Difference : simulink/Discrete/Difference  ICPrevInput=0.0  OutMin=[]  OutMax=[]  OutDataType=fixdt(1, 16)  OutScaling=2^-10  DoSatur=off
  Discrete Impulse1 : dspsrcs4/Discrete  Impulse  Delay=0  SampleTime=1  FrameSample=1  dataType=double  isSigned=on  wordLen=16  udDataType=sfix(16)  fracBitsMode=Best precision  numFracBits=15  OutDataTypeStr=double  LastOutDataTypeStr=double
  Product3 : Product  RndMeth=Zero
  Total3 : Sum  Inputs=+-
  Delta : Outport
  wires:
  Total3/1 -> Delta/1
  In1/1 -> Product3/1, Difference/1
  Product3/1 -> Total3/2
  Discrete Impulse1/1 -> Product3/2
  Difference/1 -> Total3/1

== system Duke_Simulink_13a/Passivos1/Outros Passivos/Modified Difference ==
  In1 : Inport
  Difference : simulink/Discrete/Difference  ICPrevInput=0.0  OutMin=[]  OutMax=[]  OutDataType=fixdt(1, 16)  OutScaling=2^-10  DoSatur=off
  Discrete Impulse1 : dspsrcs4/Discrete  Impulse  Delay=0  SampleTime=1  FrameSample=1  dataType=double  isSigned=on  wordLen=16  udDataType=sfix(16)  fracBitsMode=Best precision  numFracBits=15  OutDataTypeStr=double  LastOutDataTypeStr=double
  Product3 : Product  RndMeth=Zero
  Total3 : Sum  Inputs=+-
  Delta : Outport
  wires:
  Total3/1 -> Delta/1
  In1/1 -> Product3/1, Difference/1
  Product3/1 -> Total3/2
  Discrete Impulse1/1 -> Product3/2
  Difference/1 -> Total3/1
